simulink model "DYN_04"  (R2018b)
settings: Solver=FixedStepAuto  StartTime=0.0  StopTime=30  FixedStep=0.01  RelTol=1e-3
(part 14 of 14)

== matlab function DYN_04/Data ==
  data: m output; L output; Pic output; I output
function [m,L,Pic,I] = DATA_6DOF()
a1=0.075; a2=0.270; a3=0.090; d1=0.335; d4=0.295; d7=0.08;
m1 = 5.6511; m2 = 4.6061; m3 = 4.2963; m4 = 1.9151; m5 = 0.3399; m6 = 0.0714;
m = [m1 m2 m3 m4 m5 m6];
L = [a1 a2 a3 d1 d4 d7];
% Pic = zeros(6,3);
% I = zeros(6,6);
Pic = [0.0373,  -0.0076,   0.1064;
       0.1127,   0.0065,   0.0648;
       0.0447,   0.0125,  -0.0554;
       0.0006,   0.0052,   0.1068;
            0,   0.0062,   0.0195;
     -0.00001,  0.00001,  0.01126];

% I1 = [ 0.0320,  -0.0017,   0.0093;
%       -0.0017,   0.0364,  -0.0018;
%        0.0093,  -0.0018,   0.0334];
I1 = [0.0320, 0.0364, 0.0334, 0.0017, 0.0018, -0.0093];
% I2 = [ 0.0099,   0.0008,  -0.0002;
%        0.0008,   0.0646,   0.0002;
%       -0.0002,   0.0002,   0.0684];
I2 = [0.0099, 0.0646, 0.0684, -0.0008, -0.0002, 0.0002];
% I3 = [ 0.0176,    0.001,   0.0007;
%         0.001,   0.0195,   0.0002;
%        0.0007,   0.0002,    0.024];
I3 = [0.0176, 0.0195, 0.024, -0.001, -0.0002, -0.0007];
% I4 =  [  0.009,        0,        0;
%              0,   0.0081,   0.0002;
%              0,   0.0002,   0.0037];
I4 = [0.009, 0.0081, 0.0037, -0, -0.0002, -0];
% I5 = [ 0.0003,        0,        0;
%             0,   0.0002,        0;
%             0,        0,   0.0003];
I5 = [0.0003, 0.0002, 0.0003, 0, 0, 0];
% I6 = [ 0.00002,        0,        0;
%              0,  0.00002,        0;
%              0,        0,  0.00003];
I6 = [0.00002, 0.0002, 0.0003, 0, 0, 0];
I = [I1; I2; I3; I4; I5; I6];

== matlab function DYN_04/CTC ==
  data: the input; dthe input; the_r input; to output; dthe_r input; ddthe_r input; M input; C input; G input
function to = fcn(the,dthe,the_r,dthe_r,ddthe_r,M,C,G)
%% Control:
% Controler parameters
% % with noise

% without noise
ld1 = 18;
ld2 = 30;
ld3 = 18;
ld4 = 34;
% 24 27
ld5 = 10;
ld6 = 10;
Kp = diag([ld1^2,ld2^2,ld3^2,ld4^2,5*ld5^2,1.5*ld6^2]);
Kv = 2*diag([ld1,ld2,ld3,ld4,ld5,ld6]);

% Designed sliding mode control
E = the_r - the;
dE = dthe_r - dthe;
alpha = M;
beta = C*dthe + G;
dto = ddthe_r + Kv*dE + Kp*E;
to = alpha*dto + beta;

== matlab function DYN_04/MATLAB Function ==
  data: u input; y output
function y = fcn(u)

if u >=10 && u<10.1
    y = 100;
elseif u >=11 && u<11.1
    y = -50;
else
    y = 0;
end

== matlab function DYN_04/MATLAB Function1 ==
  data: u input; y output
function y = fcn(u)

if u >=20 && u<20.1
    y = 300;
elseif u >=21 && u<21.1
    y = -300;
else
    y = 0;
end

== matlab function DYN_04/MATLAB Function2 ==
  data: u input; y output
function y = fcn(u)

if u >=5 && u<5.1
    y = 300;
elseif u >=6 && u<6.1
    y = -300;
else
    y = 0;
end
